simulink model "plant_block_swing_catch_working_v0"  (R2013a)
settings: Solver=ode1  StartTime=0.0  StopTime=420  RelTol=1e-3
undefined symbols (not defined in the file or in its folder): magnitude
libraries: simulink x23
settings Model: SimulationMode=external  ExtModeTrigDuration=50000  Creator=Dro  LastModifiedBy=s4357594
settings DataIOCC: LimitDataPoints=off  SignalLoggingSaveFormat=ModelDataLogs  SignalLoggingName=sigsOut
settings OptimizationCC: ExpressionDepthLimit=2147483647  InitFltsAndDblsToZero=on
settings DebuggingCC: SaveWithParameterizedLinksMsg=none  SignalResolutionControl=TryResolveAllWithWarning  SolverPrmCheckMsg=none  MultiTaskDSMMsg=warning  MultiTaskCondExecSysMsg=none  FcnCallInpInsideContextMsg=UseLocalSettings  StrictBusMsg=None
settings RTWCC: SystemTargetFile=rtwin.tlc  TemplateMakefile=rtwin.tmf  Description=Real-Time Windows Target  ProcessScript=rtwin_make_rtw_hook  IncludeERTFirstTime=on
settings RTWinTargetCC: TargetFcnLib=ansi_tfl_tmw.mat  TargetLibSuffix=_rtwin.lib  TargetPreCompLibLocation=C:\Program Files\MATLAB\R2013a\toolbox\rtw\targets\rtwin\lib\win64  CodeReplacementLibrary=ANSI_C  ModelReferenceCompliant=off  CompOptLevelCompliant=off  RTWinDir=C:/PROGRA~1/MATLAB/R2013a/toolbox/rtw/targets/rtwin  TargetArch=win64

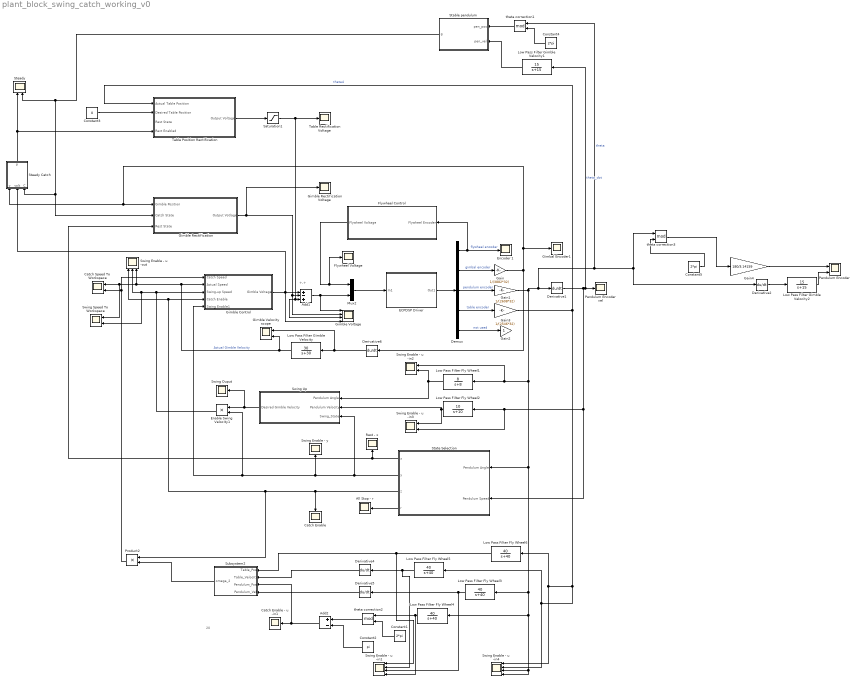
== system plant_block_swing_catch_working_v0 ==
  note: +-+
  note: 20
  Add1 : Sum  Inputs=+-+
  Add2 : Sum  Inputs=+-
  All Stop - r : Scope
      settings: YMin=-10  YMax=10  SaveName=ScopeData33
  Catch Enable : Scope
      settings: YMin=0.95  YMax=1.05  SaveName=ScopeData12
  Catch Enable - u -in1 : Scope
      settings: YMin=-3.5  YMax=3.5  SaveName=ScopeData26
  Catch Speed To Workspace : Scope  NumInputPorts=2
      settings: YMin=-10~-5  YMax=10~5  SaveName=Catch_Speed
  Constant1 : Constant  Value=2*pi
  Constant2 : Constant  Value=pi
  Constant3 : Constant  Value=0
  Constant4 : Constant  Value=2*pi
  Constant5 : Constant  Value=2*pi
  Demux : Demux  Outputs=5
  Derivative{1..2,4..6} (5 alike) : Derivative
  ECPDSP Driver : Subsystem  mask{BaseAddr='0xC000', STime=0.008, TimeOutPer=500, HWAccess=on}
      mask prompts: BaseAddr "Base I/O Address"; STime "Sample Time (Sec)"; TimeOutPer "Timeout Period (500 ~ 2000)"; HWAccess "Hardware Access"
      mask Display: color('black');disp('ECPDSP Driver\n upto\n 4 Encs(ADC Channels)\n and 2 Dacs')
  Enable Swing Velocity1 : Product
  Encoder 1 : Scope
      settings: YMin=1.5e+06  YMax=8.5e+06  SaveName=ScopeData3
  Flywheel Control : Subsystem
  Flywheel Voltage : Scope
      settings: YMin=30400  YMax=33600  SaveName=ScopeData6
  Gain : Gain  Gain=1/(3882*32)
  Gain1 : Gain  Gain=1/(2608*32)
  Gain2 : Gain
  Gain3 : Gain  Gain=1/(2546*32)
  Gain4 : Gain  Gain=180/3.14159
  Gimbal Encoder1 : Scope
      settings: YMin=-0.25  YMax=3.25  SaveName=ScopeData9
  Gimble Control : Subsystem
  Gimble Rectification : Subsystem
  Gimble Rectification Voltage : Scope
      settings: YMin=-467.5  YMax=-415  SaveName=ScopeData42
  Gimble Velocity scope : Scope  NumInputPorts=2
      settings: YMin=-10~-5  YMax=10~5  SaveName=ScopeData32
  Gimble Voltage : Scope  NumInputPorts=4
      settings: TimeRange=4.21022074346109  YMin=-460.8~459.7~-1~-1  YMax=-459.7~460.8~1~1  SaveName=ScopeData23
  Low Pass Filter Fly Wheel1 : TransferFcn  Numerator=[8]  Denominator=[1 8]
  Low Pass Filter Fly Wheel2 : TransferFcn  Numerator=[10]  Denominator=[1 10]
  Low Pass Filter Fly Wheel{3..6} (4 alike) : TransferFcn  Numerator=[40]  Denominator=[1 40]
  Low Pass Filter Gimble Velocity : TransferFcn  Numerator=[30]  Denominator=[1 30]
  Low Pass Filter Gimble Velocity1 : TransferFcn  Numerator=[15]  Denominator=[1 15]
  Low Pass Filter Gimble Velocity2 : TransferFcn  Numerator=[15]  Denominator=[1 15]
  Mux2 : Mux  Inputs=2
  Pendulum Encoder : Scope  NumInputPorts=2
      settings: YMin=0.08447~-1.4e-94  YMax=0.0933616~-1.33061e-110  SaveName=ScopeData5
  Pendulum Encoder vel : Scope
      settings: YMin=-0.08  YMax=0.15  SaveName=ScopeData19
  Product2 : Product
  Rest - x : Scope
      settings: YMin=-10  YMax=10  SaveName=ScopeData15
  Saturation1 : Saturate  UpperLimit=23500  LowerLimit=-23500
  Stable pendulum : Stateflow chart  TreatAsAtomicUnit=on
  State Selection : Subsystem
  Steady : Scope  NumInputPorts=2
      settings: YMin=30400~-5  YMax=33600~5  SaveName=ScopeData43
  Steady Catch : Stateflow chart  TreatAsAtomicUnit=on
  Subsystem2 : Subsystem
  Swing Enable - u -in1 : Scope  NumInputPorts=4
      settings: YMin=-10~-5~-5~-5  YMax=10~5~5~5  SaveName=ScopeData38
  Swing Enable - u -in2 : Scope  NumInputPorts=2
      settings: YMin=-10~-5  YMax=10~5  SaveName=ScopeData30
  Swing Enable - u -in3 : Scope  NumInputPorts=2
      settings: YMin=-10~-5  YMax=10~5  SaveName=ScopeData31
  Swing Enable - u -in4 : Scope  NumInputPorts=4
      settings: YMin=-0.5~-0.5~9.33~9.33  YMax=0.7~0.7~9.5~9.5  SaveName=ScopeData2
  Swing Enable - u -out : Scope  NumInputPorts=3
      settings: YMin=-10~-5~-5  YMax=10~5~5  SaveName=ScopeData18
  Swing Enable - y : Scope
      settings: YMin=-10  YMax=10  SaveName=ScopeData16
  Swing Ouput : Scope
      settings: YMin=-10  YMax=10  SaveName=ScopeData17
  Swing Speed To Workspace : Scope  NumInputPorts=2
      settings: YMin=-10~-5  YMax=10~5  SaveName=Swing_Speed
  Swing Up : Subsystem
  Table Position Rectification : Subsystem
  Table Rectification Voltage : Scope
      settings: YMin=-467.5  YMax=-415  SaveName=ScopeData29
  theta correction1 : Math  Operator=mod  SaturateOnIntegerOverflow=on
  theta correction2 : Math  Operator=mod  SaturateOnIntegerOverflow=on
  theta correction3 : Math  Operator=mod  SaturateOnIntegerOverflow=on
  wires:
  ECPDSP Driver/1(Out1) -> Demux/1
  Demux/1 -> Flywheel Control/1(Flywheel Encoder), Encoder 1/1  "flywheel encoder"
  Demux/2 -> Gain/1  "gimbal encoder"
  Demux/3 -> Gain1/1  "pendulum encoder"
  Demux/4 -> Gain3/1  "table encoder"
  Demux/5 -> Gain2/1  "not used"
  Derivative1/1 -> Pendulum Encoder vel/1, Low Pass Filter Gimble Velocity1/1, State Selection/2(Pendulum Speed), Swing Enable - u -in3/2, Low Pass Filter Fly Wheel2/1  "theta_dot"
  Gain1/1 -> theta correction3/1, Derivative2/1, theta correction1/1, Derivative1/1, Swing Enable - u -in4/3, Swing Enable - u -in4/4, Low Pass Filter Fly Wheel4/1, Low Pass Filter Fly Wheel3/1, State Selection/1(Pendulum Angle), Swing Enable - u -in2/1, Low Pass Filter Fly Wheel1/1  "theta"
  Swing Up/1(Desired Gimble Velocity) -> Swing Ouput/1, Enable Swing Velocity1/1
  Subsystem2/1(omega_2) -> Product2/2
  theta correction2/1 -> Add2/1
  Add2/1 -> Subsystem2/3(Pendulum_Pos), Catch Enable - u -in1/1
  Mux2/1 -> ECPDSP Driver/1(In1)
  Derivative4/1 -> Subsystem2/2(Table_Velocity)
  Constant1/1 -> theta correction2/2
  Constant2/1 -> Add2/2
  Derivative6/1 -> Low Pass Filter Gimble Velocity/1, Gimble Velocity scope/1
  Low Pass Filter Fly Wheel2/1 -> Swing Up/2(Pendulum Velocity), Swing Enable - u -in3/1
  Low Pass Filter Gimble Velocity/1 -> Gimble Velocity scope/2, Swing Enable - u -out/3, Catch Speed To Workspace/1, Swing Speed To Workspace/1, Gimble Control/2(Actual Speed)  "Actual Gimble Velocity"
  Low Pass Filter Fly Wheel1/1 -> Swing Enable - u -in2/2, Swing Up/1(Pendulum Angle)
  Flywheel Control/1(Flywheel Voltage) -> Flywheel Voltage/1, Mux2/1
  State Selection/2(y) -> Enable Swing Velocity1/2, Gimble Control/5(Swing Enable1), Swing Enable - y/1, Swing Up/3(Swing_State)
  Gain3/1 -> Table Position Rectification/1(Actual Table Position), Swing Enable - u -in4/1, Low Pass Filter Fly Wheel6/1, Swing Enable - u -in4/2, Low Pass Filter Fly Wheel5/1  "theta4"
  Low Pass Filter Fly Wheel4/1 -> theta correction2/1, Swing Enable - u -in1/4
  Derivative5/1 -> Subsystem2/4(Pendulum_Vel)
  Low Pass Filter Fly Wheel3/1 -> Derivative5/1, Swing Enable - u -in1/3
  Low Pass Filter Fly Wheel5/1 -> Swing Enable - u -in1/2, Derivative4/1
  Low Pass Filter Fly Wheel6/1 -> Swing Enable - u -in1/1, Subsystem2/1(Table_Pos)
  Gimble Control/1(Gimble Voltage) -> Gimble Voltage/4, Steady Catch/2(volt), Add1/1
  Add1/1 -> Mux2/2, Gimble Voltage/1
  Product2/1 -> Catch Speed To Workspace/2, Gimble Control/1(Catch Speed)
  Enable Swing Velocity1/1 -> Gimble Control/3(Swing-up Speed), Swing Speed To Workspace/2, Swing Enable - u -out/2
  State Selection/1(x) -> Gimble Rectification/3(Rest State), Rest - x/1
  State Selection/4(r) -> All Stop - r/1
  Gimble Rectification/1(Output Votlage) -> Gimble Voltage/2, Add1/2, Gimble Rectification Voltage/1
  Constant3/1 -> Table Position Rectification/2(Desired Table Position)
  Steady Catch/1(p) -> Table Position Rectification/4(Rect Enabled), Steady/1
  State Selection/3(z) -> Gimble Control/4(Catch Enable), Swing Enable - u -out/1, Product2/1, Catch Enable/1
  Table Position Rectification/1(Output Voltage) -> Saturation1/1
  Saturation1/1 -> Table Rectification Voltage/1, Gimble Voltage/3, Add1/3
  Stable pendulum/1(g) -> Steady/2, Gimble Rectification/2(Catch State), Steady Catch/3(C)
  Low Pass Filter Gimble Velocity1/1 -> Stable pendulum/2(pen_vel)
  Gain4/1 -> Pendulum Encoder/1
  Low Pass Filter Gimble Velocity2/1 -> Pendulum Encoder/2
  Derivative2/1 -> Low Pass Filter Gimble Velocity2/1
  Gain/1 -> Steady Catch/1(v), Gimble Rectification/1(Gimble Position), Gimbal Encoder1/1, Derivative6/1
  theta correction1/1 -> Stable pendulum/1(pen_pos)
  Constant4/1 -> theta correction1/2
  theta correction3/1 -> Gain4/1
  Constant5/1 -> theta correction3/2
  ? -> Table Position Rectification/3(Rest State)

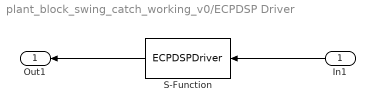
== system plant_block_swing_catch_working_v0/ECPDSP Driver ==
  In1 : Inport
  S-Function : S-Function  FunctionName=ECPDSPDriver  Parameters=BaseAddr,STime,TimeOutPer,HWAccess  EnableBusSupport=off
  Out1 : Outport
  wires:
  In1/1 -> S-Function/1
  S-Function/1 -> Out1/1

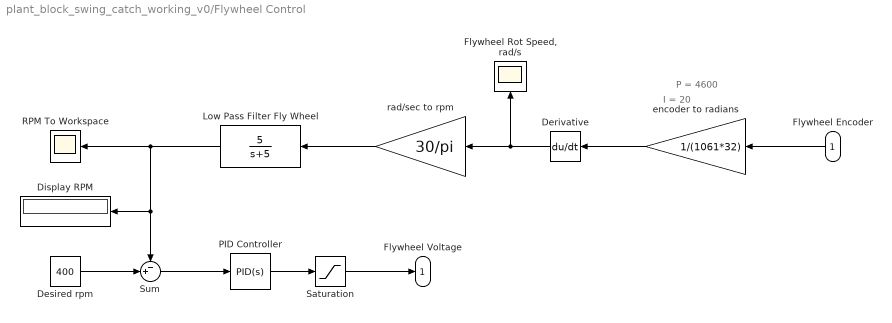
== system plant_block_swing_catch_working_v0/Flywheel Control ==
  note: I = 20
  note: P = 4600
  Flywheel Encoder : Inport
  Derivative : Derivative
  Desired rpm : Constant  Value=400
  Display RPM : Display
  "Flywheel Rot Speed, rad/s" : Scope
      settings: SaveName=ScopeData4
  Low Pass Filter Fly Wheel : TransferFcn  Numerator=[5]  Denominator=[1 5]
  PID Controller : simulink/Continuous/PID Controller  Controller=PID  TimeDomain=Continuous-time  SampleTime=1  IntegratorMethod=Forward Euler  FilterMethod=Forward Euler  Form=Parallel  P=4600  I=20  D=0  N=100  InitialConditionSource=internal  InitialConditionForIntegrator=0  InitialConditionForFilter=0  ExternalReset=none  LimitOutput=off  UpperSaturationLimit=inf  LowerSaturationLimit=-inf  LinearizeAsGain=on  AntiWindupMode=none  Kb=1  TrackingMode=off  Kt=1  PParamMin=[]  PParamMax=[]  IParamMin=[]  IParamMax=[]  DParamMin=[]  DParamMax=[]  NParamMin=[]  NParamMax=[]  KbParamMin=[]  KbParamMax=[]  KtParamMin=[]  KtParamMax=[]  POutMin=[]  POutMax=[]  IOutMin=[]  IOutMax=[]  DOutMin=[]  DOutMax=[]  NOutMin=[]  NOutMax=[]  KbOutMin=[]  KbOutMax=[]  KtOutMin=[]  KtOutMax=[]  IntegratorOutMin=[]  IntegratorOutMax=[]  FilterOutMin=[]  FilterOutMax=[]  SumOutMin=[]  SumOutMax=[]  SumI1OutMin=[]  SumI1OutMax=[]  SumI2OutMin=[]  SumI2OutMax=[]  SumI3OutMin=[]  SumI3OutMax=[]  SumDOutMin=[]  SumDOutMax=[]  SaturationOutMin=[]  SaturationOutMax=[]  IntegratorContinuousStateAttributes=''  IntegratorStateMustResolveToSignalObject=off  IntegratorRTWStateStorageClass=Auto  FilterContinuousStateAttributes=''  FilterStateMustResolveToSignalObject=off  FilterRTWStateStorageClass=Auto
  RPM To Workspace : Scope
      settings: YMin=401.6  YMax=403.9  SaveName=Flywheel_RPM
  Saturation : Saturate  UpperLimit=32000  LowerLimit=-32000
  Sum : Sum  Inputs=-+|
  encoder to radians : Gain  Gain=1/(1061*32)
  rad/sec to rpm : Gain  Gain=30/pi
  Flywheel Voltage : Outport
  wires:
  Saturation/1 -> Flywheel Voltage/1
  Sum/1 -> PID Controller/1
  Desired rpm/1 -> Sum/2
  rad/sec to rpm/1 -> Low Pass Filter Fly Wheel/1
  Derivative/1 -> "Flywheel Rot Speed, rad/s"/1, rad/sec to rpm/1
  encoder to radians/1 -> Derivative/1
  Low Pass Filter Fly Wheel/1 -> Sum/1, Display RPM/1, RPM To Workspace/1
  PID Controller/1 -> Saturation/1
  Flywheel Encoder/1 -> encoder to radians/1

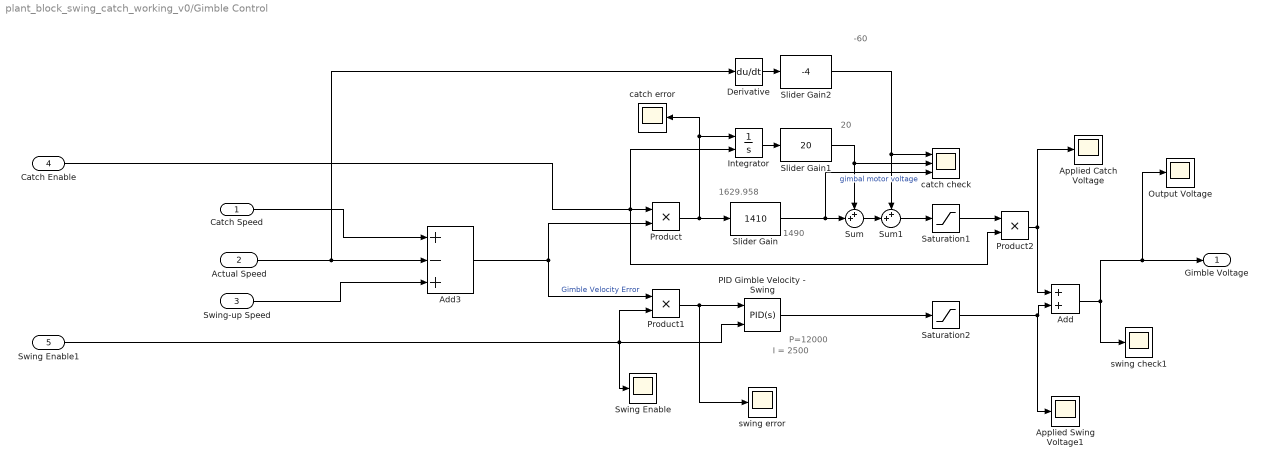
== system plant_block_swing_catch_working_v0/Gimble Control ==
  note: 1490
  note: I = 2500
  note: P=12000
  note: -60
  note: 20
  note: 1629.958
  Catch Speed : Inport
  Actual Speed : Inport  Port=2
  Swing-up Speed : Inport  Port=3
  Catch Enable : Inport  Port=4
  Swing Enable1 : Inport  Port=5
  Add : Sum
  Add3 : Sum  Inputs=+-+
  Applied Catch Voltage : Scope
      settings: SaveName=ScopeData14
  Applied Swing Voltage1 : Scope
      settings: SaveName=ScopeData22
  Derivative : Derivative
  Integrator : Integrator  ExternalReset=falling
  Output Voltage : Scope
      settings: SaveName=ScopeData37
  PID Gimble Velocity - Swing : simulink/Continuous/PID Controller  Controller=PID  TimeDomain=Continuous-time  SampleTime=1  IntegratorMethod=Forward Euler  FilterMethod=Forward Euler  Form=Parallel  P=10000  I=2500  D=0  N=100  InitialConditionSource=internal  InitialConditionForIntegrator=0  InitialConditionForFilter=0  ExternalReset=falling  LimitOutput=off  UpperSaturationLimit=inf  LowerSaturationLimit=-inf  LinearizeAsGain=on  AntiWindupMode=none  Kb=1  TrackingMode=off  Kt=1  PParamMin=[]  PParamMax=[]  IParamMin=[]  IParamMax=[]  DParamMin=[]  DParamMax=[]  NParamMin=[]  NParamMax=[]  KbParamMin=[]  KbParamMax=[]  KtParamMin=[]  KtParamMax=[]  POutMin=[]  POutMax=[]  IOutMin=[]  IOutMax=[]  DOutMin=[]  DOutMax=[]  NOutMin=[]  NOutMax=[]  KbOutMin=[]  KbOutMax=[]  KtOutMin=[]  KtOutMax=[]  IntegratorOutMin=[]  IntegratorOutMax=[]  FilterOutMin=[]  FilterOutMax=[]  SumOutMin=[]  SumOutMax=[]  SumI1OutMin=[]  SumI1OutMax=[]  SumI2OutMin=[]  SumI2OutMax=[]  SumI3OutMin=[]  SumI3OutMax=[]  SumDOutMin=[]  SumDOutMax=[]  SaturationOutMin=[]  SaturationOutMax=[]  IntegratorContinuousStateAttributes=''  IntegratorStateMustResolveToSignalObject=off  IntegratorRTWStateStorageClass=Auto  FilterContinuousStateAttributes=''  FilterStateMustResolveToSignalObject=off  FilterRTWStateStorageClass=Auto
  Product : Product
  Product1 : Product
  Product2 : Product
  Saturation1 : Saturate  UpperLimit=50000  LowerLimit=-50000
  Saturation2 : Saturate  UpperLimit=23500  LowerLimit=-23500
  Slider Gain : simulink/Math Operations/Slider Gain  low=0  gain=1410  high=2000
  Slider Gain1 : simulink/Math Operations/Slider Gain  low=0  gain=20  high=2000
  Slider Gain2 : simulink/Math Operations/Slider Gain  low=-200  gain=-4  high=0
  Sum : Sum  Inputs=++|
  Sum1 : Sum  Inputs=++|
  Swing Enable : Scope
      settings: SaveName=ScopeData10
  catch check : Scope  NumInputPorts=3
      settings: TimeRange=420  YMin=-2250~-1~-1  YMax=2750~1~1  SaveName=ScopeData21
  catch error : Scope
      settings: SaveName=ScopeData24
  swing check1 : Scope
      settings: SaveName=ScopeData27
  swing error : Scope
      settings: SaveName=ScopeData25
  Gimble Voltage : Outport
  wires:
  Add3/1 -> Product1/1, Product/2  "Gimble Velocity Error"
  Add/1 -> Output Voltage/1, Gimble Voltage/1, swing check1/1
  PID Gimble Velocity - Swing/1 -> Saturation2/1
  Product/1 -> Slider Gain/1, Integrator/1, catch error/1
  Catch Speed/1 -> Add3/1
  Catch Enable/1 -> Integrator/2, Product2/2, Product/1
  Product1/1 -> swing error/1, PID Gimble Velocity - Swing/1
  Swing-up Speed/1 -> Add3/3
  Saturation2/1 -> Applied Swing Voltage1/1, Add/2
  Integrator/1 -> Slider Gain1/1
  Slider Gain1/1 -> catch check/2, Sum/1
  Slider Gain/1 -> catch check/3, Sum/2  "gimbal motor voltage"
  Swing Enable1/1 -> Swing Enable/1, PID Gimble Velocity - Swing/2, Product1/2
  Sum/1 -> Sum1/2
  Sum1/1 -> Saturation1/1
  Slider Gain2/1 -> catch check/1, Sum1/1
  Derivative/1 -> Slider Gain2/1
  Actual Speed/1 -> Derivative/1, Add3/2
  Saturation1/1 -> Product2/1
  Product2/1 -> Add/1, Applied Catch Voltage/1

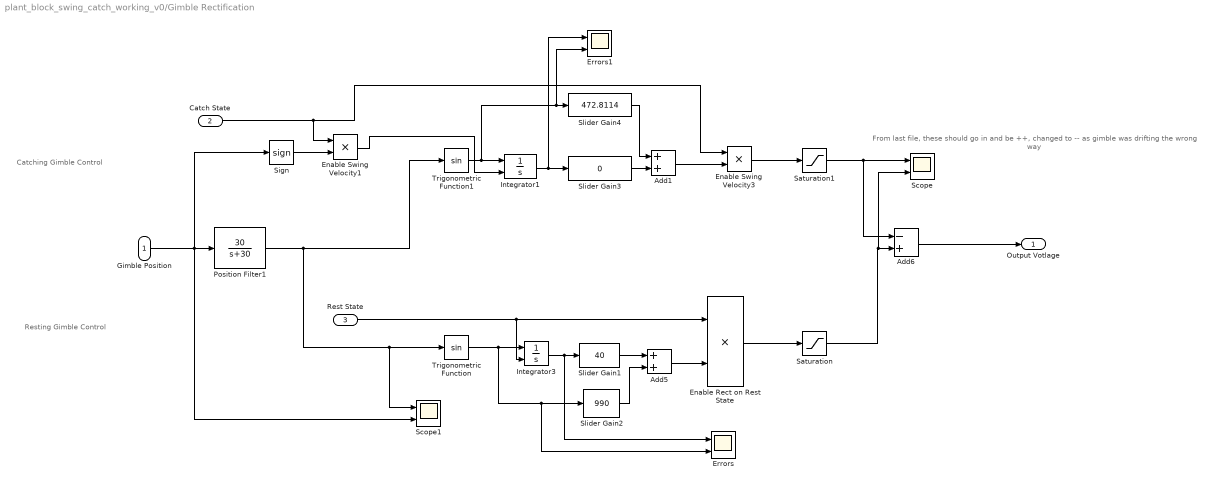
== system plant_block_swing_catch_working_v0/Gimble Rectification ==
  note: Catching Gimble Control
  note: Resting Gimble Control
  note: From last file, these should go in and be ++, changed to -- as gimble was drifting the wrong way
  Gimble Position : Inport
  Catch State : Inport  Port=2
  Rest State : Inport  Port=3
  Add1 : Sum
  Add5 : Sum
  Add6 : Sum  Inputs=-+
  Enable Rect on Rest State : Product
  Enable Swing Velocity1 : Product
  Enable Swing Velocity3 : Product
  Errors : Scope  NumInputPorts=2
      settings: YMin=-6.2~-0.135  YMax=-5.75~-0.105  SaveName=ScopeData44
  Errors1 : Scope  NumInputPorts=2
      settings: YMin=-5.25~-0.553494  YMax=-3.25~-0.553494  SaveName=ScopeData11
  Integrator1 : Integrator  ExternalReset=either
  Integrator3 : Integrator  ExternalReset=falling
  Position Filter1 : TransferFcn  Numerator=[30]  Denominator=[1 30]
  Saturation : Saturate  UpperLimit=40000  LowerLimit=-40000
  Saturation1 : Saturate  UpperLimit=2500  LowerLimit=-2500
  Scope : Scope  NumInputPorts=2
      settings: YMin=-1~-65.5  YMax=1~-54.5  SaveName=ScopeData41
  Scope1 : Scope  NumInputPorts=2
      settings: YMin=0.2775~0.2775  YMax=0.305~0.305  SaveName=ScopeData45
  Sign : Signum
  Slider Gain1 : simulink/Math Operations/Slider Gain  low=0  gain=40  high=2000
  Slider Gain2 : simulink/Math Operations/Slider Gain  low=0  gain=990  high=2000
  Slider Gain3 : simulink/Math Operations/Slider Gain  low=0  gain=0  high=2000
  Slider Gain4 : simulink/Math Operations/Slider Gain  low=0  gain=472.8114  high=1800
  Trigonometric Function : Trigonometry
  Trigonometric Function1 : Trigonometry
  Output Votlage : Outport
  wires:
  Add5/1 -> Enable Rect on Rest State/2
  Slider Gain1/1 -> Add5/1
  Slider Gain2/1 -> Add5/2
  Enable Rect on Rest State/1 -> Saturation/1
  Gimble Position/1 -> Position Filter1/1, Scope1/2, Sign/1
  Enable Swing Velocity3/1 -> Saturation1/1
  Add6/1 -> Output Votlage/1
  Saturation/1 -> Scope/2, Add6/2
  Saturation1/1 -> Scope/1, Add6/1
  Position Filter1/1 -> Trigonometric Function/1, Scope1/1, Trigonometric Function1/1
  Integrator3/1 -> Slider Gain1/1, Errors/1
  Trigonometric Function/1 -> Integrator3/1, Errors/2, Slider Gain2/1
  Rest State/1 -> Integrator3/2, Enable Rect on Rest State/1
  Slider Gain3/1 -> Add1/2
  Add1/1 -> Enable Swing Velocity3/2
  Slider Gain4/1 -> Add1/1
  Integrator1/1 -> Errors1/1, Slider Gain3/1
  Trigonometric Function1/1 -> Errors1/2, Slider Gain4/1, Integrator1/1
  Catch State/1 -> Enable Swing Velocity1/1, Enable Swing Velocity3/1
  Sign/1 -> Enable Swing Velocity1/2
  Enable Swing Velocity1/1 -> Integrator1/2

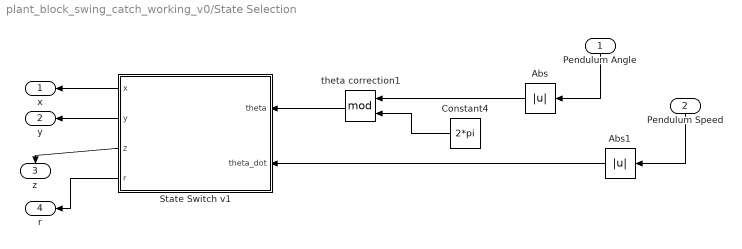
== system plant_block_swing_catch_working_v0/State Selection ==
  Pendulum Angle : Inport
  Pendulum Speed : Inport  Port=2
  Abs : Abs
  Abs1 : Abs
  Constant4 : Constant  Value=2*pi
  State Switch v1 : Stateflow chart  TreatAsAtomicUnit=on
  theta correction1 : Math  Operator=mod  SaturateOnIntegerOverflow=on
  x : Outport
  y : Outport  Port=2
  z : Outport  Port=3
  r : Outport  Port=4
  wires:
  Pendulum Angle/1 -> Abs/1
  Pendulum Speed/1 -> Abs1/1
  Abs1/1 -> State Switch v1/2(theta_dot)
  State Switch v1/2(y) -> y/1
  State Switch v1/4(r) -> r/1
  State Switch v1/1(x) -> x/1
  theta correction1/1 -> State Switch v1/1(theta)
  Constant4/1 -> theta correction1/2
  Abs/1 -> theta correction1/1
  State Switch v1/3(z) -> z/1

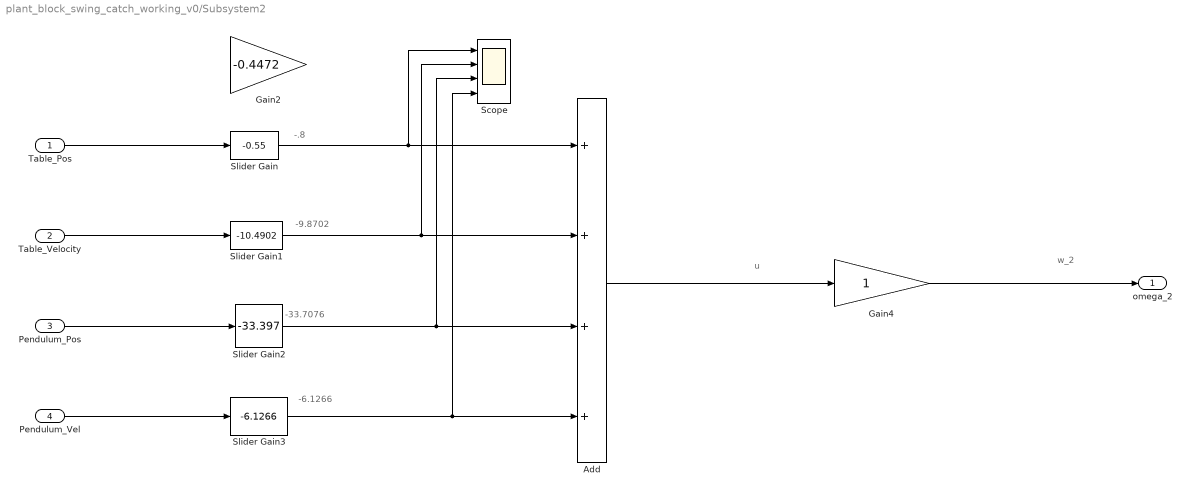
== system plant_block_swing_catch_working_v0/Subsystem2 ==
  note: -6.1266
  note: -33.7076
  note: -9.8702
  note: -.8
  note: w_2
  note: u
  Table_Pos : Inport
  Table_Velocity : Inport  Port=2
  Pendulum_Pos : Inport  Port=3
  Pendulum_Vel : Inport  Port=4
  Add : Sum  Inputs=++++
  Gain2 : Gain  Gain=-0.4472
  Gain4 : Gain
  Scope : Scope  NumInputPorts=4
      settings: YMin=-0.5~-12.5~-150~-100  YMax=1.5~12.5~150~90  SaveName=ScopeData8
  Slider Gain : simulink/Math Operations/Slider Gain  low=-20  gain=-0.55  high=5
  Slider Gain1 : simulink/Math Operations/Slider Gain  low=-30  gain=-10.4902  high=1
  Slider Gain2 : simulink/Math Operations/Slider Gain  low=-80  gain=-33.397  high=1
  Slider Gain3 : simulink/Math Operations/Slider Gain  low=-20  gain=-6.1266  high=1
  omega_2 : Outport
  wires:
  Slider Gain/1 -> Scope/1, Add/1
  Slider Gain1/1 -> Scope/2, Add/2
  Table_Pos/1 -> Slider Gain/1
  Table_Velocity/1 -> Slider Gain1/1
  Slider Gain2/1 -> Scope/3, Add/3
  Slider Gain3/1 -> Scope/4, Add/4
  Pendulum_Pos/1 -> Slider Gain2/1
  Pendulum_Vel/1 -> Slider Gain3/1
  Add/1 -> Gain4/1
  Gain4/1 -> omega_2/1

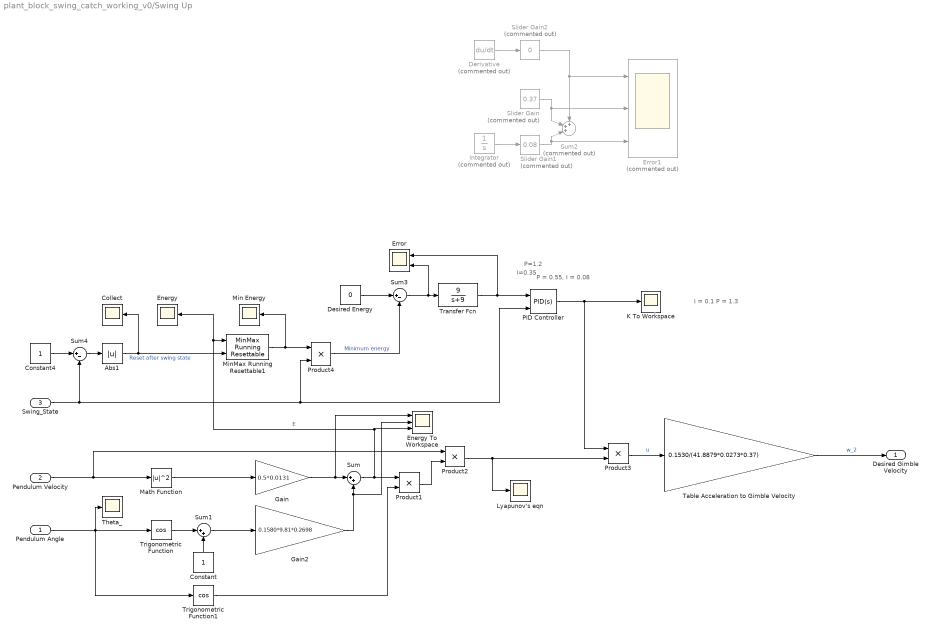
== system plant_block_swing_catch_working_v0/Swing Up ==
  note: P = 0.55, I = 0.08
  note: I=0.35
  note: P=1.2
  note: I = 0.1
      | P = 1.3
  Pendulum Angle : Inport
  Pendulum Velocity : Inport  Port=2
  Swing_State : Inport  Port=3
  Abs1 : Abs
  Collect : Scope
      settings: YMin=0.82  YMax=0.8575  SaveName=ScopeData35
  Constant : Constant
  Constant4 : Constant
  Derivative : Derivative  Commented=on
  Desired Energy : Constant  Value=0
  Energy : Scope
      settings: YMin=0.82  YMax=0.8575  SaveName=ScopeData7
  Energy To Workspace : Scope  NumInputPorts=3
      settings: YMin=-10~-5~-5  YMax=10~5~5  SaveName=Energy
  Error : Scope  NumInputPorts=2
      settings: YMin=0.82~-5  YMax=0.8575~5  SaveName=ScopeData36
  Error1 : Scope  Commented=on  NumInputPorts=3
      settings: YMin=-1~-0.09~-0.00075  YMax=1~1.38778e-17~-0.0005
  Gain : Gain  Gain=0.5*0.0131
  Gain2 : Gain  Gain=0.1580*9.81*0.2698
  Integrator : Integrator  Commented=on  ExternalReset=falling
  K To Workspace : Scope
      settings: YMin=-1.5  YMax=8.5  SaveName=Swing_Gain
  Lyapunov's eqn : Scope
      settings: YMin=-10  YMax=10
  Math Function : Math  Operator=magnitude^2  SaturateOnIntegerOverflow=on
  Min Energy : Scope
      settings: YMin=0.82  YMax=0.8575  SaveName=ScopeData34
  MinMax Running Resettable1 : simulink/Math Operations/MinMax Running Resettable  Function=min  vinit=0.85
  PID Controller : simulink/Continuous/PID Controller  Controller=PID  TimeDomain=Continuous-time  SampleTime=1  IntegratorMethod=Forward Euler  FilterMethod=Forward Euler  Form=Parallel  P=0.48  I=0.06  D=0  N=100  InitialConditionSource=internal  InitialConditionForIntegrator=0  InitialConditionForFilter=0  ExternalReset=falling  LimitOutput=off  UpperSaturationLimit=inf  LowerSaturationLimit=-inf  LinearizeAsGain=on  AntiWindupMode=none  Kb=1  TrackingMode=off  Kt=1  PParamMin=[]  PParamMax=[]  IParamMin=[]  IParamMax=[]  DParamMin=[]  DParamMax=[]  NParamMin=[]  NParamMax=[]  KbParamMin=[]  KbParamMax=[]  KtParamMin=[]  KtParamMax=[]  POutMin=[]  POutMax=[]  IOutMin=[]  IOutMax=[]  DOutMin=[]  DOutMax=[]  NOutMin=[]  NOutMax=[]  KbOutMin=[]  KbOutMax=[]  KtOutMin=[]  KtOutMax=[]  IntegratorOutMin=[]  IntegratorOutMax=[]  FilterOutMin=[]  FilterOutMax=[]  SumOutMin=[]  SumOutMax=[]  SumI1OutMin=[]  SumI1OutMax=[]  SumI2OutMin=[]  SumI2OutMax=[]  SumI3OutMin=[]  SumI3OutMax=[]  SumDOutMin=[]  SumDOutMax=[]  SaturationOutMin=[]  SaturationOutMax=[]  IntegratorContinuousStateAttributes=''  IntegratorStateMustResolveToSignalObject=off  IntegratorRTWStateStorageClass=Auto  FilterContinuousStateAttributes=''  FilterStateMustResolveToSignalObject=off  FilterRTWStateStorageClass=Auto
  Product{1..4} (4 alike) : Product
  Slider Gain : simulink/Math Operations/Slider Gain  Commented=on  low=0  gain=0.37  high=1
  Slider Gain1 : simulink/Math Operations/Slider Gain  Commented=on  low=0  gain=0.08  high=0.5
  Slider Gain2 : simulink/Math Operations/Slider Gain  Commented=on  low=-0.5  gain=0  high=0
  Sum : Sum  Inputs=|++
  Sum1 : Sum  Inputs=|++
  Sum2 : Sum  Commented=on  Inputs=+++|
  Sum3 : Sum  Inputs=|+-
  Sum4 : Sum  Inputs=|+-
  Table Acceleration to Gimble Velocity : Gain  Gain=0.1530/(41.8879*0.0273*0.37)
  Theta_ : Scope
      settings: YMin=-10  YMax=10  SaveName=ScopeData28
  Transfer Fcn : TransferFcn  Numerator=[9]  Denominator=[1 9]
  Trigonometric Function : Trigonometry  Operator=cos
  Trigonometric Function1 : Trigonometry  Operator=cos
  Desired Gimble Velocity : Outport
  wires:
  Pendulum Velocity/1 -> Math Function/1, Product2/1
  Math Function/1 -> Gain/1
  Gain/1 -> Energy To Workspace/1, Sum/1
  Product3/1 -> Table Acceleration to Gimble Velocity/1  "u"
  Trigonometric Function/1 -> Sum1/1
  Constant/1 -> Sum1/2
  Sum1/1 -> Gain2/1
  Sum/1 -> Energy To Workspace/3, Energy/1, MinMax Running Resettable1/1, Product1/1  "E"
  Trigonometric Function1/1 -> Product1/2
  Product1/1 -> Product2/2
  Gain2/1 -> Sum/2, Energy To Workspace/2
  Product2/1 -> Product3/2, Lyapunov's eqn/1
  Table Acceleration to Gimble Velocity/1 -> Desired Gimble Velocity/1  "w_2"
  Pendulum Angle/1 -> Theta_/1, Trigonometric Function1/1, Trigonometric Function/1
  Sum3/1 -> Error/2, Transfer Fcn/1
  Desired Energy/1 -> Sum3/1
  Product4/1 -> Sum3/2  "Minimum energy"
  Swing_State/1 -> PID Controller/2, Product4/2, Sum4/2
  Constant4/1 -> Sum4/1
  Sum4/1 -> Abs1/1
  MinMax Running Resettable1/1 -> Product4/1, Min Energy/1
  Transfer Fcn/1 -> Error/1, PID Controller/1
  Abs1/1 -> Collect/1, MinMax Running Resettable1/2  "Reset after swing state"
  Integrator/1 -> Slider Gain1/1
  Slider Gain/1 -> Sum2/2, Error1/2
  Slider Gain2/1 -> Sum2/1, Error1/1
  Slider Gain1/1 -> Error1/3, Sum2/3
  Derivative/1 -> Slider Gain2/1
  PID Controller/1 -> K To Workspace/1, Product3/1

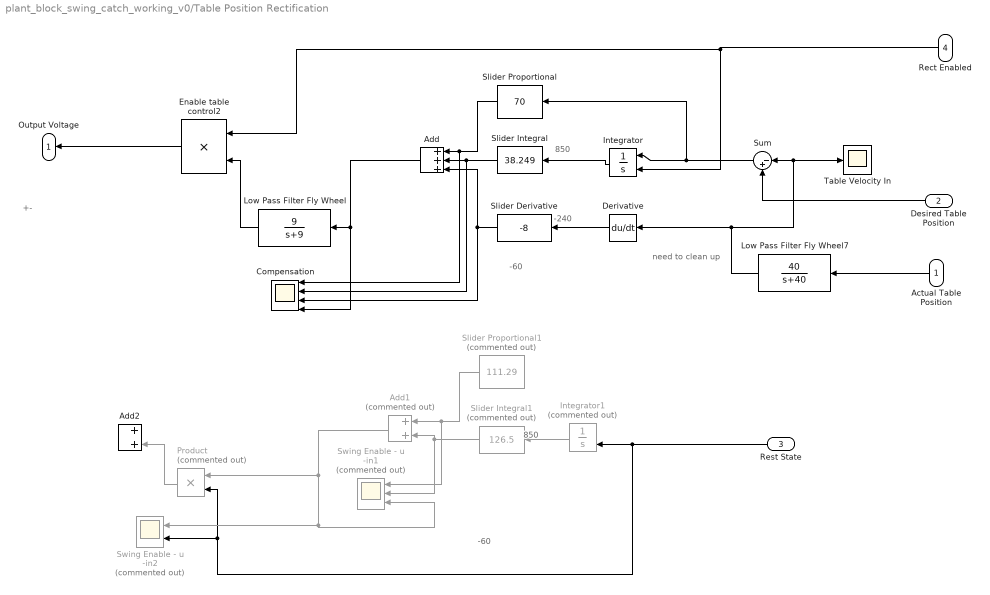
== system plant_block_swing_catch_working_v0/Table Position Rectification ==
  note: +-
  note: -60
  note: -240
  note: 850
  note: need to clean up
  note: -60
  note: 850
  Actual Table Position : Inport
  Desired Table Position : Inport  Port=2
  Rest State : Inport  Port=3
  Rect Enabled : Inport  Port=4
  Add : Sum  Inputs=+++
  Add1 : Sum  Commented=on
  Add2 : Sum
  Compensation : Scope  NumInputPorts=4
      settings: YMin=-200~48~-1~-150  YMax=150~68~1~225  SaveName=ScopeData40
  Derivative : Derivative
  Enable table control2 : Product
  Integrator : Integrator  ExternalReset=falling
  Integrator1 : Integrator  Commented=on  ExternalReset=falling
  Low Pass Filter Fly Wheel : TransferFcn  Numerator=[9]  Denominator=[1 9]
  Low Pass Filter Fly Wheel7 : TransferFcn  Numerator=[40]  Denominator=[1 40]
  Product : Product  Commented=on
  Slider Derivative : simulink/Math Operations/Slider Gain  low=-200  gain=-8  high=0
  Slider Integral : simulink/Math Operations/Slider Gain  low=0  gain=38.249  high=1000
  Slider Integral1 : simulink/Math Operations/Slider Gain  Commented=on  low=0  gain=126.5  high=5000
  Slider Proportional : simulink/Math Operations/Slider Gain  low=0  gain=70  high=500
  Slider Proportional1 : simulink/Math Operations/Slider Gain  Commented=on  low=0  gain=111.29  high=5000
  Sum : Sum  Inputs=|-+
  Swing Enable - u -in1 : Scope  Commented=on  NumInputPorts=3
      settings: YMin=2.15~11~13  YMax=2.475~13.75~16.25  SaveName=ScopeData46
  Swing Enable - u -in2 : Scope  Commented=on  NumInputPorts=2
      settings: YMin=6.7~0.95  YMax=9~1.05  SaveName=ScopeData47
  Table Velocity In : Scope
      settings: YMin=-0.016  YMax=0.003  SaveName=ScopeData13
  Output Voltage : Outport
  wires:
  Actual Table Position/1 -> Low Pass Filter Fly Wheel7/1
  Desired Table Position/1 -> Sum/2
  Slider Integral/1 -> Compensation/2, Add/2
  Slider Derivative/1 -> Compensation/3, Add/3
  Slider Proportional/1 -> Compensation/1, Add/1
  Integrator/1 -> Slider Integral/1
  Derivative/1 -> Slider Derivative/1
  Add/1 -> Compensation/4, Low Pass Filter Fly Wheel/1
  Low Pass Filter Fly Wheel7/1 -> Table Velocity In/1, Sum/1, Derivative/1
  Rest State/1 -> Product/2, Swing Enable - u -in2/2, Integrator1/2
  Slider Integral1/1 -> Add1/2, Swing Enable - u -in1/2
  Slider Proportional1/1 -> Swing Enable - u -in1/1, Add1/1
  Integrator1/1 -> Slider Integral1/1
  Add1/1 -> Product/1, Swing Enable - u -in1/3, Swing Enable - u -in2/1
  Product/1 -> Add2/2
  Low Pass Filter Fly Wheel/1 -> Enable table control2/2
  Rect Enabled/1 -> Integrator/2, Enable table control2/1
  Sum/1 -> Integrator/1, Slider Proportional/1
  Enable table control2/1 -> Output Voltage/1

== stateflow chart plant_block_swing_catch_working_v0/Steady Catch ==
  state En_On
    entry:
    p = 0;
  state En_Off
    entry:
    p = 1;
  (default) -> En_On
  En_On -> En_Off : [abs(v) < 0.08 & abs(volt) < 4000 & C > 0]
  En_Off -> En_On : [abs(v) > 0.08& abs(volt) > 4000 & C < 1]
  data: p output double; v input; volt input; C input

== stateflow chart plant_block_swing_catch_working_v0/State Selection/State Switch v1 ==
  state Swing
    entry:
    x = 0,
    y = 1,
    z = 0,
    r = 0;
  state Rest
    entry:
    x = 1,
    y = 0,
    z = 0;
    r = 0;
  state Catch
    entry:
    x = 0,
    y = 0,
    z = 1;
    r = 0;
  state ReSwing
    entry:
    x = 0,
    y = 0,
    z = 0;
    r = 1;
  (default) -> Rest
  Rest -> Swing : [theta > 0.12 & theta_dot > 0.12]
  ReSwing -> Swing : [theta_dot < 2 & (theta < (pi/4) | theta > (2*pi- pi/4))]
  Swing -> Rest [order 2] : [theta < 0.12 & theta_dot < 0.12]
  Swing -> Catch [order 1] : [(3.14 - (3.14/10)) < theta & theta < (3.14 + (3.14/10))]
  Catch -> ReSwing [order 1] : [theta_dot > 6 & theta > (pi-pi/8) & theta < (pi+pi/8)]
  Catch -> ReSwing [order 2] : [theta < (3.14 - (3.14/10)) | theta > (3.14 + (3.14/10))]
  data: x output; y output; z output; theta input; theta_dot input; r output

== stateflow chart plant_block_swing_catch_working_v0/Stable pendulum ==
  state Gimble
    entry:
    g = 0;
  state Gimble_go
    entry:
    g = 1;
  Gimble -> Gimble_go : [(abs(pen_vel) < 0.1) & (abs(pen_pos) > (177*3.14/180) & abs(pen_pos) < (183*3.14/180))]
  (default) -> Gimble
  Gimble_go -> Gimble : [(abs(pen_vel) > 0.1) & (abs(pen_pos) < (177*3.14/180) | abs(pen_pos) > (183*3.14/180))]
  data: pen_pos input; pen_vel input; g output double
